simulink model "model_example"  (R2019b)
settings: Solver=FixedStepDiscrete  StartTime=0.0  StopTime=1000  RelTol=1e-3  EnableMultiTasking=on
values from neighbouring files (symbols this model uses):
  b = 2    [beispielsystem.m]    (also in init.m = 0.8; init_loesung.m = xdash0+xdash0*pp; model_dsc.m = block.DialogPrm(3).data)
  Delta = 1    [beispielsystem.m]    (also in init.m; init_loesung.m = 0.01; model_dsc.m = block.DialogPrm(1).data)
  z0 = [0;0]    [init.m]
settings Model: Creator=schauer  LastModifiedBy=schauer
settings DataIOCC: LimitDataPoints=on  ReturnWorkspaceOutputs=off
settings OptimizationCC: LifeSpan=inf
settings DebuggingCC: AllowSymbolicDim=off  SFUnexpectedBacktrackingDiag=warning  SFNoUnconditionalDefaultTransitionDiag=warning  SFExecutionAtInitializationDiag=none  ArithmeticOperatorsInVariantConditions=warning
settings ModelReferenceCC: PropagateSignalLabelsOutOfModel=off
settings SFSimCC: SimUseLocalCustomCode=off  CustomCodeUndefinedFunction=UseInterfaceOnly
settings RTWCC: RTWUseLocalCustomCode=off
settings CodeAppCC: StateflowObjectComments=on
settings GRTTargetCC: TargetLangStandard=C89/C90 (ANSI)
settings ConfigComp: CovMetricSettings=dw  CovHtmlReporting=on  CovSaveCumulativeToWorkspaceVar=on  CovSaveSingleToWorkspaceVar=on  CovExternalEMLEnable=off

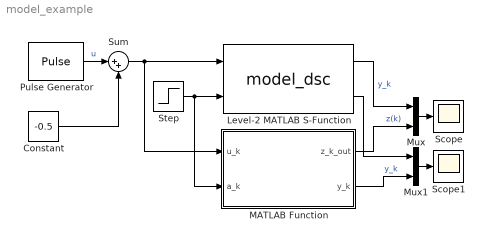
== system model_example ==
  Constant : Constant  Value=-0.5
  Level-2 MATLAB S-Function : M-S-Function  FunctionName=model_dsc  Parameters=Delta,z0,b
  MATLAB Function : MATLAB Function  TreatAsAtomicUnit=on  SystemSampleTime=Delta
  Mux : Mux  Inputs=2
  Mux1 : Mux  Inputs=2
  Pulse Generator : DiscretePulseGenerator  Period=100  PulseWidth=50
  Scope : Scope
  Scope1 : Scope
  Step : Step  Time=500  Before=0.5  After=0.2  SampleTime=1
  Sum : Sum  Inputs=|++
  wires:
  Level-2 MATLAB S-Function/1 -> Mux/1  "y_k"
  Step/1 -> MATLAB Function/2(a_k), Level-2 MATLAB S-Function/2
  Mux/1 -> Scope/1
  MATLAB Function/1(z_k_out) -> Mux/2  "z(k)"
  Pulse Generator/1 -> Sum/1  "u"
  Sum/1 -> MATLAB Function/1(u_k), Level-2 MATLAB S-Function/1
  Constant/1 -> Sum/2
  Mux1/1 -> Scope1/1
  MATLAB Function/2(y_k) -> Mux1/2  "y_k"
  Level-2 MATLAB S-Function/2 -> Mux1/1

== matlab function model_example/MATLAB Function ==
  data: u_k input; a_k input; z_k_out output; z0 parameter; b parameter; y_k output
function [z_k_out,y_k] = fcn(u_k, a_k, z0, b)

%initialize states (variables to be stored)
persistent  z_k 
if isempty(z_k) 
    z_k= z0;
end
%Update states and calulate output 
z_kp1=[0.4*z_k(1) + 0.2*z_k(2);
       b*z_k(1) + a_k*z_k(2)+u_k];
y_k    = 0.6*z_k(1)+0.2*z_k(2)+0.4*randn(1);
z_k_out = z_k;           
%Store states
z_k = z_kp1;
